simulink model "shower"  (Simulink 2.20)
settings: Solver=ode45  StartTime=0  StopTime=10000  MaxStep=0.1  RelTol=1e-3  AbsTol=1e-3
PreLoadFcn:
  | fisMatrix=readfis('shower'); k=1;
settings Model: SaveTime=off  SaveOutput=off  ConsistencyChecking=off  RTWPlaceOutputsASAP=off  RTWTemplateMakefile=grt_vc.tmf

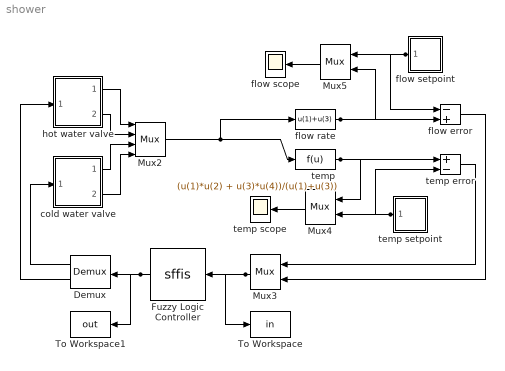
== system shower ==
  Demux : Demux  Orientation=left  Outputs=2
  Fuzzy Logic Controller : S-Function  Orientation=left  FunctionName=sffis  Parameters=fismatrix  PortCounts=[]  SFunctionModules=sfsup  mask(FIS){@1=fisMatrix}
      mask prompts: @1 "FIS Matrix:"
      mask help: FIS
      mask init:
      | fismatrix = @1;
      mask Help: Fuzzy Inference System
      mask Display: plot(0, -0.3, 6, -0.3, 0, 1.2, 6, 1.2, [0 6], [0 0], [1 2 3],[0 1 0],[2 3 4],[0 1 0],[3 4 5],[0 1 0])
  Mux2 : Mux  Inputs=4
  Mux3 : Mux  Orientation=left  Inputs=2
  Mux4 : Mux  Orientation=left  Inputs=2
  Mux5 : Mux  Orientation=left  Inputs=2
  To Workspace : ToWorkspace  VariableName=in  SampleTime=0
      settings: Buffer=1000
  To Workspace1 : ToWorkspace  VariableName=out  SampleTime=0
      settings: Buffer=1000
  cold water valve : Subsystem
  flow error : Sum  Inputs=-+
  flow scope : Scope
      settings: TickLabels=on  TimeRange=50.000000  YMin=-1.000000  YMax=1.000000  SaveToWorkspace=off  SaveName=ScopeData
  flow setpoint : Subsystem  Orientation=left
  flow rate : Fcn  Expr=u(1)+u(3)
  hot water valve : Subsystem
  temp : Fcn  Expr=(u(1)*u(2) + u(3)*u(4))/(u(1)+u(3))
  temp error : Sum  Inputs=+-
  temp scope : Scope
      settings: TickLabels=on  TimeRange=50.000000  YMin=-30.000000  YMax=30.000000  SaveToWorkspace=off  SaveName=ScopeData
  temp setpoint : Subsystem  Orientation=left
  wires:
  cold water valve/1(out_1) -> Mux2/3
  hot water valve/1(out_1) -> Mux2/1
  hot water valve/2(out_2) -> Mux2/2
  cold water valve/2(out_2) -> Mux2/4
  Demux/1 -> cold water valve/1(in_1)
  Demux/2 -> hot water valve/1(in_1)
  Mux3/1 -> Fuzzy Logic Controller/1, To Workspace/1
  temp error/1 -> Mux3/1
  flow error/1 -> Mux3/2
  Fuzzy Logic Controller/1 -> Demux/1, To Workspace1/1
  Mux2/1 -> flow rate/1, temp/1
  Mux4/1 -> temp scope/1
  temp/1 -> temp error/1, Mux4/1
  temp setpoint/1(out_1) -> temp error/2, Mux4/2
  Mux5/1 -> flow scope/1
  flow rate/1 -> flow error/2, Mux5/2
  flow setpoint/1(out_1) -> flow error/1, Mux5/1

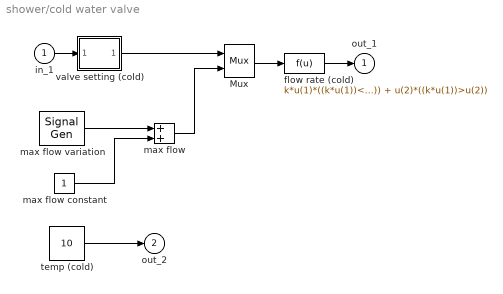
== system shower/cold water valve ==
  in_1 : Inport  Port=1  PortWidth=-1  SampleTime=-1
  Mux : Mux  Inputs=2
  flow rate (cold) : Fcn  Expr=k*u(1)*((k*u(1))<=u(2)) + u(2)*((k*u(1))>u(2))
  max flow : Sum  Inputs=++
  max flow constant : Constant  Value=1
  max flow variation : SignalGenerator  WaveForm=sine  Amplitude=0.000000  Frequency=0.101325  Units=rad/sec
  temp (cold) : Constant  Value=10
  valve setting (cold) : Subsystem  mask(Limited Integrator.){@1=0.001, @2=2, @3=0.1}
      mask prompts: @1 "Lower bound:"; @2 "Upper bound:"; @3 "Initial condition:"
      mask help: Limited Integrator
      mask init:
      | lower_limit=@1;upper_limit=@2;X0=@3;
      mask Help: Implements a limited integrator with \nan expression of the form:\n\nif(x<=lb and u<0) or (x>=ub and u>0)\n   xdot=0\nelse\n   xdot=u
      mask Display: plot(-1,-0.2,3.5,1.2,[0.05,1,2,2.9],[0,0,1,1]);disp(' 1/s    ')
  out_1 : Outport  Port=1  InitialOutput=0
  out_2 : Outport  Port=2  InitialOutput=0
  wires:
  max flow/1 -> Mux/2
  max flow variation/1 -> max flow/1
  max flow constant/1 -> max flow/2
  temp (cold)/1 -> out_2/1
  flow rate (cold)/1 -> out_1/1
  in_1/1 -> valve setting (cold)/1(Inport)
  Mux/1 -> flow rate (cold)/1
  valve setting (cold)/1(Outport) -> Mux/1

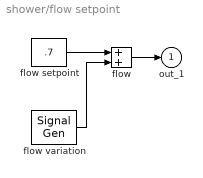
== system shower/flow setpoint ==
  flow : Sum  Inputs=++
  flow setpoint : Constant  Value=.7
  flow variation : SignalGenerator  WaveForm=square  Amplitude=0.200000  Frequency=0.300000  Units=rad/sec
  out_1 : Outport  Port=1  InitialOutput=0
  wires:
  flow setpoint/1 -> flow/1
  flow variation/1 -> flow/2
  flow/1 -> out_1/1

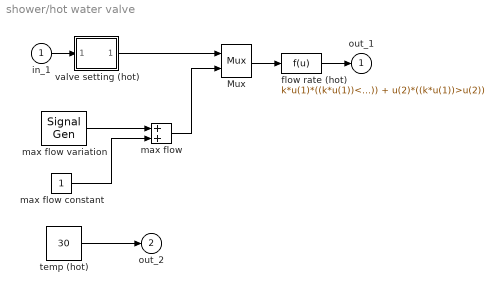
== system shower/hot water valve ==
  in_1 : Inport  Port=1  PortWidth=-1  SampleTime=-1
  Mux : Mux  Inputs=2
  flow rate (hot) : Fcn  Expr=k*u(1)*((k*u(1))<=u(2)) + u(2)*((k*u(1))>u(2))
  max flow : Sum  Inputs=++
  max flow constant : Constant  Value=1
  max flow variation : SignalGenerator  WaveForm=sine  Amplitude=0.000000  Frequency=0.300000  Units=rad/sec
  temp (hot) : Constant  Value=30
  valve setting (hot) : Subsystem  mask(Limited Integrator.){@1=0.001, @2=2, @3=.1}
      mask prompts: @1 "Lower bound:"; @2 "Upper bound:"; @3 "Initial condition:"
      mask help: Limited Integrator
      mask init:
      | lower_limit=@1;upper_limit=@2;X0=@3;
      mask Help: Implements a limited integrator with \nan expression of the form:\n\nif(x<=lb and u<0) or (x>=ub and u>0)\n   xdot=0\nelse\n   xdot=u
      mask Display: plot(-1,-0.2,3.5,1.2,[0.05,1,2,2.9],[0,0,1,1]);disp(' 1/s    ')
  out_1 : Outport  Port=1  InitialOutput=0
  out_2 : Outport  Port=2  InitialOutput=0
  wires:
  valve setting (hot)/1(Outport) -> Mux/1
  Mux/1 -> flow rate (hot)/1
  in_1/1 -> valve setting (hot)/1(Inport)
  flow rate (hot)/1 -> out_1/1
  temp (hot)/1 -> out_2/1
  max flow constant/1 -> max flow/2
  max flow variation/1 -> max flow/1
  max flow/1 -> Mux/2

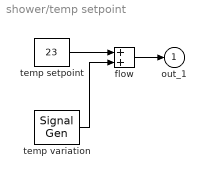
== system shower/temp setpoint ==
  flow : Sum  Inputs=++
  temp setpoint : Constant  Value=23
  temp variation : SignalGenerator  WaveForm=square  Amplitude=4.000000  Frequency=0.214320  Units=rad/sec
  out_1 : Outport  Port=1  InitialOutput=0
  wires:
  flow/1 -> out_1/1
  temp variation/1 -> flow/2
  temp setpoint/1 -> flow/1

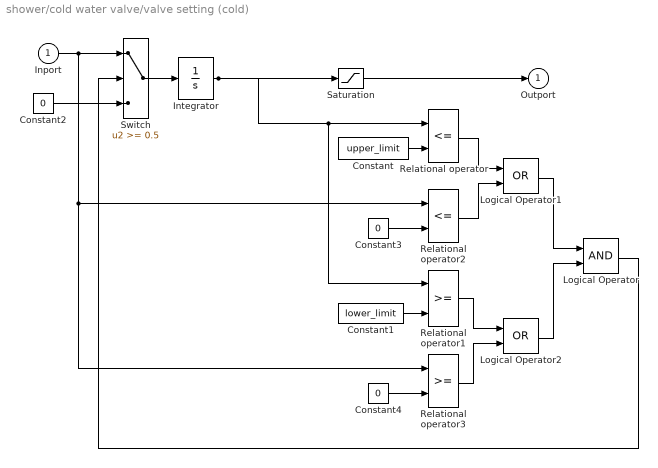
== system shower/cold water valve/valve setting (cold) ==
  Inport : Inport  Port=1  PortWidth=-1  SampleTime=-1
  Constant : Constant  Value=upper_limit
  Constant1 : Constant  Value=lower_limit
  Constant2 : Constant  Value=0
  Constant3 : Constant  Value=0
  Constant4 : Constant  Value=0
  Integrator : Integrator  ExternalReset=none  InitialConditionSource=internal  InitialCondition=X0  LimitOutput=off  UpperSaturationLimit=inf  LowerSaturationLimit=-inf  ShowSaturationPort=off  ShowStatePort=off  AbsoluteTolerance=auto
  Logical Operator : Logic  Operator=AND  Inputs=2
  Logical Operator1 : Logic  Operator=OR  Inputs=2
  Logical Operator2 : Logic  Operator=OR  Inputs=2
  Relational operator : RelationalOperator  Operator=<=
  Relational operator1 : RelationalOperator  Operator=>=
  Relational operator2 : RelationalOperator  Operator=<=
  Relational operator3 : RelationalOperator  Operator=>=
  Saturation : Saturate  UpperLimit=upper_limit  LowerLimit=lower_limit
  Switch : Switch  Threshold=0.5
  Outport : Outport  Port=1  InitialOutput=0
  wires:
  Constant4/1 -> Relational operator3/2
  Constant3/1 -> Relational operator2/2
  Logical Operator2/1 -> Logical Operator/2
  Relational operator3/1 -> Logical Operator2/2
  Relational operator1/1 -> Logical Operator2/1
  Logical Operator1/1 -> Logical Operator/1
  Relational operator2/1 -> Logical Operator1/2
  Relational operator/1 -> Logical Operator1/1
  Constant2/1 -> Switch/3
  Logical Operator/1 -> Switch/2
  Constant1/1 -> Relational operator1/2
  Constant/1 -> Relational operator/2
  Switch/1 -> Integrator/1
  Inport/1 -> Switch/1, Relational operator2/1, Relational operator3/1
  Integrator/1 -> Relational operator1/1, Relational operator/1, Saturation/1
  Saturation/1 -> Outport/1

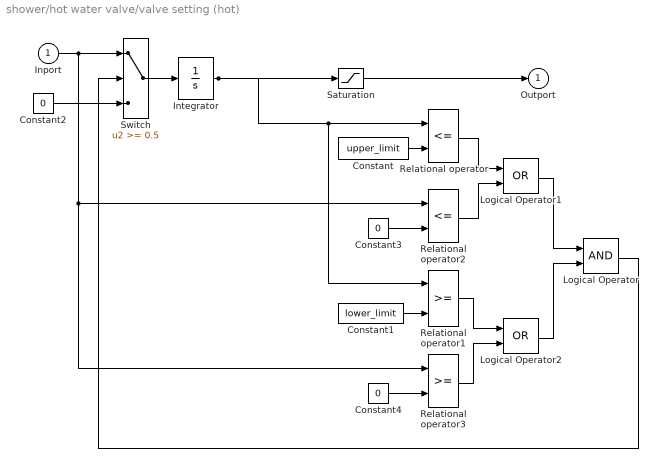
== system shower/hot water valve/valve setting (hot) ==
  Inport : Inport  Port=1  PortWidth=-1  SampleTime=-1
  Constant : Constant  Value=upper_limit
  Constant1 : Constant  Value=lower_limit
  Constant2 : Constant  Value=0
  Constant3 : Constant  Value=0
  Constant4 : Constant  Value=0
  Integrator : Integrator  ExternalReset=none  InitialConditionSource=internal  InitialCondition=X0  LimitOutput=off  UpperSaturationLimit=inf  LowerSaturationLimit=-inf  ShowSaturationPort=off  ShowStatePort=off  AbsoluteTolerance=auto
  Logical Operator : Logic  Operator=AND  Inputs=2
  Logical Operator1 : Logic  Operator=OR  Inputs=2
  Logical Operator2 : Logic  Operator=OR  Inputs=2
  Relational operator : RelationalOperator  Operator=<=
  Relational operator1 : RelationalOperator  Operator=>=
  Relational operator2 : RelationalOperator  Operator=<=
  Relational operator3 : RelationalOperator  Operator=>=
  Saturation : Saturate  UpperLimit=upper_limit  LowerLimit=lower_limit
  Switch : Switch  Threshold=0.5
  Outport : Outport  Port=1  InitialOutput=0
  wires:
  Saturation/1 -> Outport/1
  Inport/1 -> Switch/1, Relational operator2/1, Relational operator3/1
  Switch/1 -> Integrator/1
  Constant/1 -> Relational operator/2
  Constant1/1 -> Relational operator1/2
  Logical Operator/1 -> Switch/2
  Constant2/1 -> Switch/3
  Relational operator/1 -> Logical Operator1/1
  Relational operator2/1 -> Logical Operator1/2
  Logical Operator1/1 -> Logical Operator/1
  Relational operator1/1 -> Logical Operator2/1
  Relational operator3/1 -> Logical Operator2/2
  Logical Operator2/1 -> Logical Operator/2
  Constant3/1 -> Relational operator2/2
  Constant4/1 -> Relational operator3/2
  Integrator/1 -> Saturation/1, Relational operator1/1, Relational operator/1
